simulink model "BallAndHoop"  (Simulink 9.0)
settings: Solver=ode23s  StartTime=0.0  StopTime=10  MaxStep=1e-1  RelTol=1e-3  EnableMultiTasking=on
InitFcn:
  | g = 9.81; %gravitational constant
  | 
  |  % showVR = 0; %show VR world
  | %  psi_init = 0; %initial condition
libraries: vrlib x2
CloseFcn:
  | vrclose all;
  | clear figureVR worldVR;
settings Model: SuppressorTable=22 serialization::archive 11 0 6 0 0 0 11 0  Creator=H  LastModifiedBy=ladislav
settings DataIOCC: LimitDataPoints=on  SignalLoggingSaveFormat=ModelDataLogs
settings OptimizationCC: ExpressionDepthLimit=2147483647  InitFltsAndDblsToZero=on
settings DebuggingCC: SaveWithParameterizedLinksMsg=none  SignalResolutionControl=TryResolveAllWithWarning  SolverPrmCheckMsg=warning  FcnCallInpInsideContextMsg=warning  StateNameClashWarn=warning  StrictBusMsg=Warning
settings GRTTargetCC: TargetFcnLib=ansi_tfl_tmw.mat  GeneratePreprocessorConditionals=Disable all  CombineOutputUpdateFcns=off  GRTInterface=on

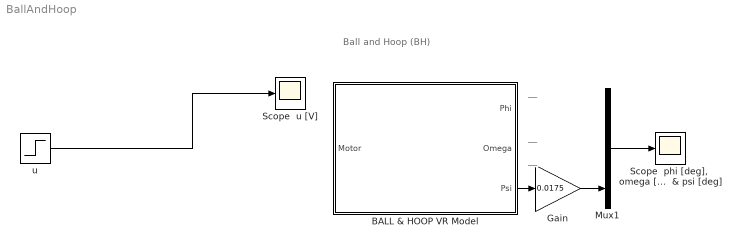
== system BallAndHoop ==
  note: Ball and Hoop (BH)
  note: __
  note: __
  note: __
  BALL & HOOP VR Model : Subsystem  mask(Ball and Hoop (BH) in laboratory K26){showVR=off, phi0=-1, brake=off}
      mask prompts: showVR "Show VirtualWorld?"; phi0 "Initial angle of the ball   psi(0)  [deg] (from the stable equil. rightwise)"; brake "Hoop brake"
      mask help: Ball and Hoop (BH) in laboratory K26 - Virtual Reality
      mask Help:
      | Ball and Hoop in laboratory K26 - Virtual Reality. <br><br>
      | 
      | 
      | This is a virtual model of the Ball and Hoop apparatus in Laboratory of automatic control
      | theory&nbsp;26 (<a href="http://support.dce.felk.cvut.cz/lab26/" target="_blank">http://support.dce.felk.cvut.cz/lab26/</a>),
      | which consists of a&nbsp;DC motor, a&nbsp;hoop and a&nbsp;ball. The&nbsp;hoop angular velocity is controlled
      | by the DC motor controller by the voltage&nbsp;<em>u</em>&nbsp;[V].  A&nbsp;metal ball is placed inside
      | the&nbsp;hoop so that it rolls in a&nbsp;groove on the&nbsp;inner periphery of the&nbsp;hoop.
      | <br><br>
      | 
      | The&nbsp;system input is the&nbsp;voltage of the&nbsp;DC motor&nbsp;<em>u</em>&nbsp;[V].
      | The&nbsp;system outputs are the&nbsp;hoop velocity&nbsp;<em>&omega;</em>&nbsp;[rot/min],
      | the&nbsp;angle of the&nbsp;hoop&nbsp;<em>&phi;</em>&nbsp;[deg] and the&nbsp;angle of
      | the&nbsp;ball&nbsp;<em>&psi;</em>&nbsp;[deg]. More information can be found on the website
      | <a href="http://support.dce.felk.cvut.cz/lab26/" target="_blank">http://support.dce.felk.cvut.cz/lab26/</a>.<br><br>
      | 
      | 
      | In the mask of the model, it can be set:
      | <ul>
      | <li>Initial angle of the ball.</li>
      | </ul><br><br>
      | 
      | 
      | Copyright: 2009, Jiri Machac, Jirka Roubal, Petr Husek.
      mask Callback showVR:
      | if strcmp('off',get_param(gcb,'showVR'))
      |     vrclose all;
      | else
      |     if exist('figureVR')==0
      |         figureVR = vrfigure;
      |     end
      |     if exist('worldVR')==0
      |         worldVR = vrworld('BallHoop_VR.WRL');
      |     end
      | 	if isvalid(figureVR)==0
      |         open(worldVR);
      |         figureVR = vrfigure(worldVR,[650 80 550 350]);
      | 	end
      | end
      mask Display:
      | image(imread('BallHoop_Image.jpg'));
      | port_label ('input',1,'u [V]');
      | port_label ('output',1,'phi [deg]');
      | port_label ('output',2,'omega [rot/min]');
      | port_label ('output',3,'psi [deg]');
  Gain : Gain  Gain=0.0175
  Mux1 : Mux  Inputs=3
  "Scope  phi [deg],  omega [rot/min]  & psi [deg]" : Scope
  Scope  u [V] : Scope
  u : Step  Time=5  Before=1  After=0.4  SampleTime=0
  wires:
  Mux1/1 -> "Scope  phi [deg],  omega [rot/min]  & psi [deg]"/1
  u/1 -> Scope  u [V]/1
  BALL & HOOP VR Model/3(Psi) -> Gain/1
  Gain/1 -> Mux1/3

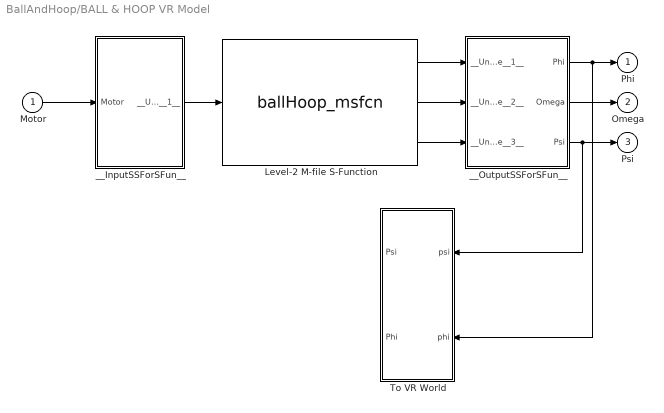
== system BallAndHoop/BALL & HOOP VR Model ==
  Motor : Inport
  Level-2 M-file S-Function : M-S-Function  FunctionName=ballHoop_msfcn  Parameters=phi0, brake
  To VR World : Subsystem
  __InputSSForSFun__ : Subsystem
  __OutputSSForSFun__ : Subsystem
  Phi : Outport  OutDataTypeStr=double  PortDimensions=1  SampleTime=[-1 0]
  Omega : Outport  Port=2  OutDataTypeStr=double  PortDimensions=1  SampleTime=[-1 0]
  Psi : Outport  Port=3  OutDataTypeStr=double  PortDimensions=1  SampleTime=[-1 0]
  wires:
  __OutputSSForSFun__/3(Psi) -> To VR World/1(psi), Psi/1
  __OutputSSForSFun__/2(Omega) -> Omega/1
  __OutputSSForSFun__/1(Phi) -> To VR World/2(phi), Phi/1
  __InputSSForSFun__/1(__UniqueOutportName__1__) -> Level-2 M-file S-Function/1
  Motor/1 -> __InputSSForSFun__/1(Motor)
  Level-2 M-file S-Function/1 -> __OutputSSForSFun__/1(__UniqueInportName__1__)
  Level-2 M-file S-Function/2 -> __OutputSSForSFun__/2(__UniqueInportName__2__)
  Level-2 M-file S-Function/3 -> __OutputSSForSFun__/3(__UniqueInportName__3__)

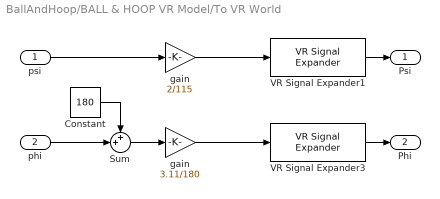
== system BallAndHoop/BALL & HOOP VR Model/To VR World ==
  psi : Inport
  phi : Inport  Port=2
  Constant : Constant  Value=180
  Sum : Sum  Inputs=++|
  VR Signal Expander1 : vrlib/VR Signal Expander  outwidth=4  outidx=[4]
      settings: SourceProductName=Simulink 3D Animation  SourceProductBaseCode=VR
  VR Signal Expander3 : vrlib/VR Signal Expander  outwidth=4  outidx=[4]
      settings: SourceProductName=Simulink 3D Animation  SourceProductBaseCode=VR
  gain : Gain  Gain=2/115
  "gain " : Gain  Gain=3.11/180
  Psi : Outport
  Phi : Outport  Port=2
  wires:
  psi/1 -> gain/1
  VR Signal Expander3/1 -> Phi/1
  VR Signal Expander1/1 -> Psi/1
  phi/1 -> Sum/2
  gain/1 -> VR Signal Expander1/1
  Constant/1 -> Sum/1
  Sum/1 -> "gain "/1
  "gain "/1 -> VR Signal Expander3/1

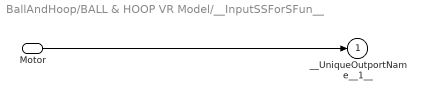
== system BallAndHoop/BALL & HOOP VR Model/__InputSSForSFun__ ==
  Motor : Inport
  __UniqueOutportName__1__ : Outport
  wires:
  Motor/1 -> __UniqueOutportName__1__/1

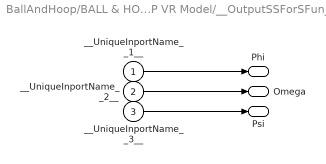
== system BallAndHoop/BALL & HOOP VR Model/__OutputSSForSFun__ ==
  __UniqueInportName__1__ : Inport
  __UniqueInportName__2__ : Inport  Port=2
  __UniqueInportName__3__ : Inport  Port=3
  Phi : Outport  OutDataTypeStr=double  PortDimensions=1  SampleTime=[-1 0]
  Omega : Outport  Port=2  OutDataTypeStr=double  PortDimensions=1  SampleTime=[-1 0]
  Psi : Outport  Port=3  OutDataTypeStr=double  PortDimensions=1  SampleTime=[-1 0]
  wires:
  __UniqueInportName__3__/1 -> Psi/1
  __UniqueInportName__2__/1 -> Omega/1
  __UniqueInportName__1__/1 -> Phi/1
